simulink model "Cell_Balancing_MATLAB_v_2025b"  (R2025b)
settings: Solver=VariableStepAuto  StopTime=3000  FixedStep=1
undefined symbols (not defined in the file): R
libraries: fl_lib x59, nesl_utility x34, batteryecm_lib x10
(part 3 of 3)

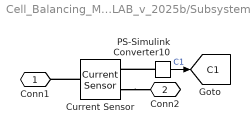
== system Cell_Balancing_MATLAB_v_2025b/Subsystem1 ==
  Current Sensor : fl_lib/Electrical/Electrical Sensors/Current Sensor
  PS-Simulink Converter10 : nesl_utility/PS-Simulink Converter  PhysicalDomain=network_engine_domain  SubClassName=ps_output  LeftPortType=input  RightPortType=output  PseudoPeriodic=off  Frequencies=[]  VectorFormat=inherit  Unit=inherit  AffineConversion=off
  Conn1 : PMIOPort  Side=Left
  Conn2 : PMIOPort  Port=2  Side=Right
  tag scope: C1=global
  wires:
  PS-Simulink Converter10/1 -> [C1]  "C1"
  connections:
  Current Sensor/LConn1 -- Conn1/RConn1
  PS-Simulink Converter10/LConn1 -- Current Sensor/RConn1
  Current Sensor/RConn2 -- Conn2/RConn1

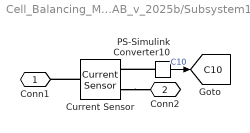
== system Cell_Balancing_MATLAB_v_2025b/Subsystem10 ==
  Current Sensor : fl_lib/Electrical/Electrical Sensors/Current Sensor
  PS-Simulink Converter10 : nesl_utility/PS-Simulink Converter  PhysicalDomain=network_engine_domain  SubClassName=ps_output  LeftPortType=input  RightPortType=output  PseudoPeriodic=off  Frequencies=[]  VectorFormat=inherit  Unit=inherit  AffineConversion=off
  Conn1 : PMIOPort  Side=Left
  Conn2 : PMIOPort  Port=2  Side=Right
  tag scope: C10=global
  wires:
  PS-Simulink Converter10/1 -> [C10]  "C10"
  connections:
  Current Sensor/LConn1 -- Conn1/RConn1
  PS-Simulink Converter10/LConn1 -- Current Sensor/RConn1
  Current Sensor/RConn2 -- Conn2/RConn1

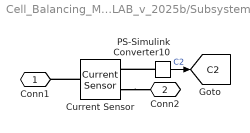
== system Cell_Balancing_MATLAB_v_2025b/Subsystem2 ==
  Current Sensor : fl_lib/Electrical/Electrical Sensors/Current Sensor
  PS-Simulink Converter10 : nesl_utility/PS-Simulink Converter  PhysicalDomain=network_engine_domain  SubClassName=ps_output  LeftPortType=input  RightPortType=output  PseudoPeriodic=off  Frequencies=[]  VectorFormat=inherit  Unit=inherit  AffineConversion=off
  Conn1 : PMIOPort  Side=Left
  Conn2 : PMIOPort  Port=2  Side=Right
  tag scope: C2=global
  wires:
  PS-Simulink Converter10/1 -> [C2]  "C2"
  connections:
  Current Sensor/LConn1 -- Conn1/RConn1
  PS-Simulink Converter10/LConn1 -- Current Sensor/RConn1
  Current Sensor/RConn2 -- Conn2/RConn1

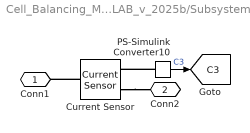
== system Cell_Balancing_MATLAB_v_2025b/Subsystem3 ==
  Current Sensor : fl_lib/Electrical/Electrical Sensors/Current Sensor
  PS-Simulink Converter10 : nesl_utility/PS-Simulink Converter  PhysicalDomain=network_engine_domain  SubClassName=ps_output  LeftPortType=input  RightPortType=output  PseudoPeriodic=off  Frequencies=[]  VectorFormat=inherit  Unit=inherit  AffineConversion=off
  Conn1 : PMIOPort  Side=Left
  Conn2 : PMIOPort  Port=2  Side=Right
  tag scope: C3=global
  wires:
  PS-Simulink Converter10/1 -> [C3]  "C3"
  connections:
  Current Sensor/LConn1 -- Conn1/RConn1
  PS-Simulink Converter10/LConn1 -- Current Sensor/RConn1
  Current Sensor/RConn2 -- Conn2/RConn1

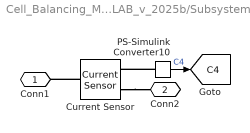
== system Cell_Balancing_MATLAB_v_2025b/Subsystem4 ==
  Current Sensor : fl_lib/Electrical/Electrical Sensors/Current Sensor
  PS-Simulink Converter10 : nesl_utility/PS-Simulink Converter  PhysicalDomain=network_engine_domain  SubClassName=ps_output  LeftPortType=input  RightPortType=output  PseudoPeriodic=off  Frequencies=[]  VectorFormat=inherit  Unit=inherit  AffineConversion=off
  Conn1 : PMIOPort  Side=Left
  Conn2 : PMIOPort  Port=2  Side=Right
  tag scope: C4=global
  wires:
  PS-Simulink Converter10/1 -> [C4]  "C4"
  connections:
  Current Sensor/LConn1 -- Conn1/RConn1
  PS-Simulink Converter10/LConn1 -- Current Sensor/RConn1
  Current Sensor/RConn2 -- Conn2/RConn1

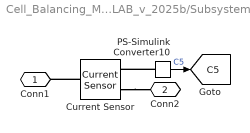
== system Cell_Balancing_MATLAB_v_2025b/Subsystem5 ==
  Current Sensor : fl_lib/Electrical/Electrical Sensors/Current Sensor
  PS-Simulink Converter10 : nesl_utility/PS-Simulink Converter  PhysicalDomain=network_engine_domain  SubClassName=ps_output  LeftPortType=input  RightPortType=output  PseudoPeriodic=off  Frequencies=[]  VectorFormat=inherit  Unit=inherit  AffineConversion=off
  Conn1 : PMIOPort  Side=Left
  Conn2 : PMIOPort  Port=2  Side=Right
  tag scope: C5=global
  wires:
  PS-Simulink Converter10/1 -> [C5]  "C5"
  connections:
  Current Sensor/LConn1 -- Conn1/RConn1
  PS-Simulink Converter10/LConn1 -- Current Sensor/RConn1
  Current Sensor/RConn2 -- Conn2/RConn1

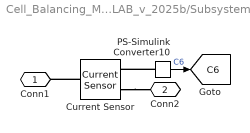
== system Cell_Balancing_MATLAB_v_2025b/Subsystem6 ==
  Current Sensor : fl_lib/Electrical/Electrical Sensors/Current Sensor
  PS-Simulink Converter10 : nesl_utility/PS-Simulink Converter  PhysicalDomain=network_engine_domain  SubClassName=ps_output  LeftPortType=input  RightPortType=output  PseudoPeriodic=off  Frequencies=[]  VectorFormat=inherit  Unit=inherit  AffineConversion=off
  Conn1 : PMIOPort  Side=Left
  Conn2 : PMIOPort  Port=2  Side=Right
  tag scope: C6=global
  wires:
  PS-Simulink Converter10/1 -> [C6]  "C6"
  connections:
  Current Sensor/LConn1 -- Conn1/RConn1
  PS-Simulink Converter10/LConn1 -- Current Sensor/RConn1
  Current Sensor/RConn2 -- Conn2/RConn1

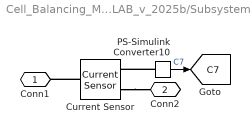
== system Cell_Balancing_MATLAB_v_2025b/Subsystem7 ==
  Current Sensor : fl_lib/Electrical/Electrical Sensors/Current Sensor
  PS-Simulink Converter10 : nesl_utility/PS-Simulink Converter  PhysicalDomain=network_engine_domain  SubClassName=ps_output  LeftPortType=input  RightPortType=output  PseudoPeriodic=off  Frequencies=[]  VectorFormat=inherit  Unit=inherit  AffineConversion=off
  Conn1 : PMIOPort  Side=Left
  Conn2 : PMIOPort  Port=2  Side=Right
  tag scope: C7=global
  wires:
  PS-Simulink Converter10/1 -> [C7]  "C7"
  connections:
  Current Sensor/LConn1 -- Conn1/RConn1
  PS-Simulink Converter10/LConn1 -- Current Sensor/RConn1
  Current Sensor/RConn2 -- Conn2/RConn1

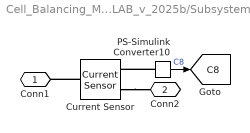
== system Cell_Balancing_MATLAB_v_2025b/Subsystem8 ==
  Current Sensor : fl_lib/Electrical/Electrical Sensors/Current Sensor
  PS-Simulink Converter10 : nesl_utility/PS-Simulink Converter  PhysicalDomain=network_engine_domain  SubClassName=ps_output  LeftPortType=input  RightPortType=output  PseudoPeriodic=off  Frequencies=[]  VectorFormat=inherit  Unit=inherit  AffineConversion=off
  Conn1 : PMIOPort  Side=Left
  Conn2 : PMIOPort  Port=2  Side=Right
  tag scope: C8=global
  wires:
  PS-Simulink Converter10/1 -> [C8]  "C8"
  connections:
  Current Sensor/LConn1 -- Conn1/RConn1
  PS-Simulink Converter10/LConn1 -- Current Sensor/RConn1
  Current Sensor/RConn2 -- Conn2/RConn1

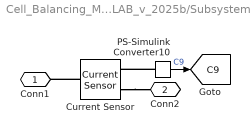
== system Cell_Balancing_MATLAB_v_2025b/Subsystem9 ==
  Current Sensor : fl_lib/Electrical/Electrical Sensors/Current Sensor
  PS-Simulink Converter10 : nesl_utility/PS-Simulink Converter  PhysicalDomain=network_engine_domain  SubClassName=ps_output  LeftPortType=input  RightPortType=output  PseudoPeriodic=off  Frequencies=[]  VectorFormat=inherit  Unit=inherit  AffineConversion=off
  Conn1 : PMIOPort  Side=Left
  Conn2 : PMIOPort  Port=2  Side=Right
  tag scope: C9=global
  wires:
  PS-Simulink Converter10/1 -> [C9]  "C9"
  connections:
  Current Sensor/LConn1 -- Conn1/RConn1
  PS-Simulink Converter10/LConn1 -- Current Sensor/RConn1
  Current Sensor/RConn2 -- Conn2/RConn1
